simulink model "simulation"  (R2022a)
settings: Solver=VariableStepAuto  StartTime=0.0  StopTime=60  FixedStep=1/1000  RelTol=1e-3
values from neighbouring files (symbols this model uses):
  b = 1    [init.m]
  bw_con = -s_cl    (= 2.66666666667)    [init.m]
  bw_eso = -s_eso    (= 26.6666666667)    [init.m]
  d = 0.1    [init.m]
  eta_init = [0 0 0 0 0]'    [init.m]
  g = 9.82    [init.m]
  L = 1    [init.m]    (also in trig2.m = 1/2 * ((m_c + m_l)*(dx^2 + dy^2 + dz^2) + m_l*L^2*(dtheta^2 )
  ldx_sat = [-5 5]    [init.m]
  ldy_sat = ldx_sat    [init.m]
  ldz_sat = ldx_sat    [init.m]
  m_c = 2.5    [init.m]
  m_l = 0.250    (= 0.25)    [init.m]
  nu_init = [0 0 -L 0 0]'    [init.m]
  xyforce = [-10 10]    [init.m]
  zforce = [-40 40]    [init.m]
libraries: slpidlib x6, SignalEditorBlockLib x1
settings Model: Creator=marti  LastModifiedBy=martin
settings DebuggingCC: UnconnectedInputMsg=warning  UnconnectedOutputMsg=warning  UnconnectedLineMsg=warning
settings RTWCC: DLArmComputeVersion=19.05

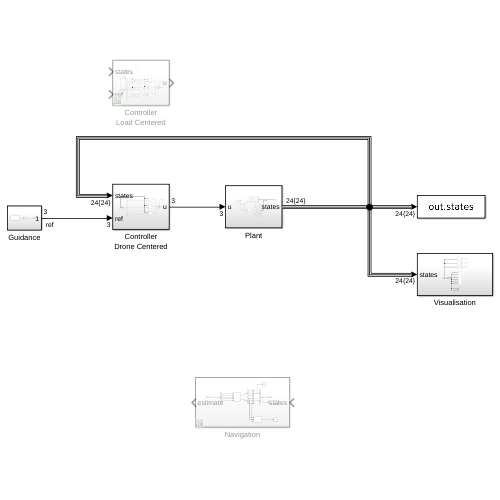
[thumbnail: Simulink's stored preview of the top-level diagram]
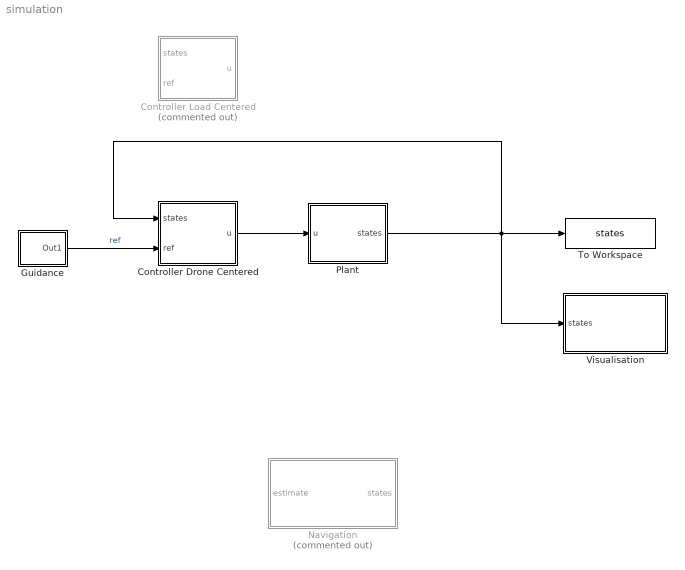
== system simulation ==
  Controller Drone Centered : Subsystem
  Controller Load Centered : Subsystem  Commented=on
  Guidance : Subsystem
  Navigation : Subsystem  Commented=on
  Plant : Subsystem
  To Workspace : ToWorkspace  VariableName=states  SaveFormat=Timeseries  SampleTime=-1
  Visualisation : Subsystem
  wires:
  Plant/1(states) -> Visualisation/1(states), Controller Drone Centered/1(states), To Workspace/1
  Controller Drone Centered/1(u) -> Plant/1(u)
  Guidance/1(Out1) -> Controller Drone Centered/2(ref)  "ref"

== system simulation/Controller Drone Centered ==
  states : Inport
  ref : Inport  Port=2
  Bus Selector : BusSelector  OutputSignals=Quadrotor.vZ
  Bus Selector1 : BusSelector  OutputSignals=Quadrotor.vY
  Bus Selector2 : BusSelector  OutputSignals=Quadrotor.vX
  Bus Selector6 : BusSelector  OutputSignals=Quadrotor.X,Quadrotor.Y,Quadrotor.Z  OutputAsBus=on
  Demux : Demux  Outputs=3
  Forces : Scope
  Mux : Mux  Inputs=3
  PID Controller : slpidlib/PID Controller  Controller=P  Form=Parallel  TimeDomain=Continuous-time  UseExternalTs=off  SampleTime=-1  IntegratorMethod=Forward Euler  FilterMethod=Forward Euler  ControllerParametersSource=internal  P=0.6  I=0  UseKiTs=off  D=0  N=100  UseFilter=on  TunerSelectOption=Transfer Function Based (PID Tuner App)  InitialConditionSource=internal  InitialConditionForIntegrator=0  InitialConditionForFilter=0  DifferentiatorICPrevScaledInput=0  ExternalReset=none  TrackingMode=off  Kt=1  LimitOutput=off  SatLimitsSource=internal  UpperSaturationLimit=inf  LowerSaturationLimit=-inf  LinearizeAsGain=on  AntiWindupMode=none  Kb=1  POutMin=[]  POutMax=[]  IOutMin=[]  IOutMax=[]  DOutMin=[]  DOutMax=[]  NOutMin=[]  NOutMax=[]  SumOutMin=[]  SumOutMax=[]  SaturationOutMin=[]  SaturationOutMax=[]  PParamMin=[]  PParamMax=[]  IParamMin=[]  IParamMax=[]  DParamMin=[]  DParamMax=[]  NParamMin=[]  NParamMax=[]  KbParamMin=[]  KbParamMax=[]  KtParamMin=[]  KtParamMax=[]  KbOutMin=[]  KbOutMax=[]  KtOutMin=[]  KtOutMax=[]  IntegratorOutMin=[]  IntegratorOutMax=[]  FilterOutMin=[]  FilterOutMax=[]  SumI1OutMin=[]  SumI1OutMax=[]  SumI2OutMin=[]  SumI2OutMax=[]  SumI3OutMin=[]  SumI3OutMax=[]  SumI4OutMin=[]  SumI4OutMax=[]  SumDOutMin=[]  SumDOutMax=[]  DifferentiatorOutMin=[]  DifferentiatorOutMax=[]  FilterDiffOutCoefMin=[]  FilterDiffOutCoefMax=[]  ReciprocalOutMin=[]  ReciprocalOutMax=[]  SumDenOutMin=[]  SumDenOutMax=[]  SumNumOutMin=[]  SumNumOutMax=[]  DivideOutMin=[]  DivideOutMax=[]  UdiffTsProdOutMin=[]  UdiffTsProdOutMax=[]  NTsProdOutMin=[]  NTsProdOutMax=[]  UintegralTsProdOutMin=[]  UintegralTsProdOutMax=[]  UngainTsProdOutMin=[]  UngainTsProdOutMax=[]  IntegratorContinuousStateAttributes=''  IntegratorStateMustResolveToSignalObject=off  IntegratorRTWStateStorageClass=Auto  FilterContinuousStateAttributes=''  FilterStateMustResolveToSignalObject=off  FilterRTWStateStorageClass=Auto  ParallelPVariant=InternalParameters  IdealPVariant=Disabled  IVariant=Disabled  DVariant=Disabled  IntegratorVariant=Disabled  SatVariant=Disabled  AWVariant=Disabled  PCopyVariant=Disabled  TRVariant=Disabled  FdbkBlocksVariant=Forward  IdealPFdbkVariant=Disabled  SatFdbkVariant=Disabled  DerivativeFilterVariant=Disabled  NVariant=Disabled  NCopyVariant=Disabled_SignalSpec  FilterICVariant=Disabled  IntegratorICVariant=Disabled  ExternalResetVariant=Disabled  TRSumVariant=Passthrough  SumFdbkVariant=Disabled  SumVariant=Passthrough_P  TsampFilterVariant=InternalTs  TsampNgainVariant=Passthrough  TsampIntegralVariant=Disabled_SignalSpec  ExternalSaturationOutDataTypeStr=Inherit: Same as second input  aMode=0
  PID Controller1 : slpidlib/PID Controller  Controller=P  Form=Parallel  TimeDomain=Continuous-time  UseExternalTs=off  SampleTime=-1  IntegratorMethod=Forward Euler  FilterMethod=Forward Euler  ControllerParametersSource=internal  P=0.6  I=0  UseKiTs=off  D=0  N=100  UseFilter=on  TunerSelectOption=Transfer Function Based (PID Tuner App)  InitialConditionSource=internal  InitialConditionForIntegrator=0  InitialConditionForFilter=0  DifferentiatorICPrevScaledInput=0  ExternalReset=none  TrackingMode=off  Kt=1  LimitOutput=off  SatLimitsSource=internal  UpperSaturationLimit=inf  LowerSaturationLimit=-inf  LinearizeAsGain=on  AntiWindupMode=none  Kb=1  POutMin=[]  POutMax=[]  IOutMin=[]  IOutMax=[]  DOutMin=[]  DOutMax=[]  NOutMin=[]  NOutMax=[]  SumOutMin=[]  SumOutMax=[]  SaturationOutMin=[]  SaturationOutMax=[]  PParamMin=[]  PParamMax=[]  IParamMin=[]  IParamMax=[]  DParamMin=[]  DParamMax=[]  NParamMin=[]  NParamMax=[]  KbParamMin=[]  KbParamMax=[]  KtParamMin=[]  KtParamMax=[]  KbOutMin=[]  KbOutMax=[]  KtOutMin=[]  KtOutMax=[]  IntegratorOutMin=[]  IntegratorOutMax=[]  FilterOutMin=[]  FilterOutMax=[]  SumI1OutMin=[]  SumI1OutMax=[]  SumI2OutMin=[]  SumI2OutMax=[]  SumI3OutMin=[]  SumI3OutMax=[]  SumI4OutMin=[]  SumI4OutMax=[]  SumDOutMin=[]  SumDOutMax=[]  DifferentiatorOutMin=[]  DifferentiatorOutMax=[]  FilterDiffOutCoefMin=[]  FilterDiffOutCoefMax=[]  ReciprocalOutMin=[]  ReciprocalOutMax=[]  SumDenOutMin=[]  SumDenOutMax=[]  SumNumOutMin=[]  SumNumOutMax=[]  DivideOutMin=[]  DivideOutMax=[]  UdiffTsProdOutMin=[]  UdiffTsProdOutMax=[]  NTsProdOutMin=[]  NTsProdOutMax=[]  UintegralTsProdOutMin=[]  UintegralTsProdOutMax=[]  UngainTsProdOutMin=[]  UngainTsProdOutMax=[]  IntegratorContinuousStateAttributes=''  IntegratorStateMustResolveToSignalObject=off  IntegratorRTWStateStorageClass=Auto  FilterContinuousStateAttributes=''  FilterStateMustResolveToSignalObject=off  FilterRTWStateStorageClass=Auto  ParallelPVariant=InternalParameters  IdealPVariant=Disabled  IVariant=Disabled  DVariant=Disabled  IntegratorVariant=Disabled  SatVariant=Disabled  AWVariant=Disabled  PCopyVariant=Disabled  TRVariant=Disabled  FdbkBlocksVariant=Forward  IdealPFdbkVariant=Disabled  SatFdbkVariant=Disabled  DerivativeFilterVariant=Disabled  NVariant=Disabled  NCopyVariant=Disabled_SignalSpec  FilterICVariant=Disabled  IntegratorICVariant=Disabled  ExternalResetVariant=Disabled  TRSumVariant=Passthrough  SumFdbkVariant=Disabled  SumVariant=Passthrough_P  TsampFilterVariant=InternalTs  TsampNgainVariant=Passthrough  TsampIntegralVariant=Disabled_SignalSpec  ExternalSaturationOutDataTypeStr=Inherit: Same as second input  aMode=0
  PID Controller2 : slpidlib/PID Controller  Controller=P  Form=Parallel  TimeDomain=Continuous-time  UseExternalTs=off  SampleTime=-1  IntegratorMethod=Forward Euler  FilterMethod=Forward Euler  ControllerParametersSource=internal  P=0.6  I=0  UseKiTs=off  D=0  N=100  UseFilter=on  TunerSelectOption=Transfer Function Based (PID Tuner App)  InitialConditionSource=internal  InitialConditionForIntegrator=0  InitialConditionForFilter=0  DifferentiatorICPrevScaledInput=0  ExternalReset=none  TrackingMode=off  Kt=1  LimitOutput=off  SatLimitsSource=internal  UpperSaturationLimit=inf  LowerSaturationLimit=-inf  LinearizeAsGain=on  AntiWindupMode=none  Kb=1  POutMin=[]  POutMax=[]  IOutMin=[]  IOutMax=[]  DOutMin=[]  DOutMax=[]  NOutMin=[]  NOutMax=[]  SumOutMin=[]  SumOutMax=[]  SaturationOutMin=[]  SaturationOutMax=[]  PParamMin=[]  PParamMax=[]  IParamMin=[]  IParamMax=[]  DParamMin=[]  DParamMax=[]  NParamMin=[]  NParamMax=[]  KbParamMin=[]  KbParamMax=[]  KtParamMin=[]  KtParamMax=[]  KbOutMin=[]  KbOutMax=[]  KtOutMin=[]  KtOutMax=[]  IntegratorOutMin=[]  IntegratorOutMax=[]  FilterOutMin=[]  FilterOutMax=[]  SumI1OutMin=[]  SumI1OutMax=[]  SumI2OutMin=[]  SumI2OutMax=[]  SumI3OutMin=[]  SumI3OutMax=[]  SumI4OutMin=[]  SumI4OutMax=[]  SumDOutMin=[]  SumDOutMax=[]  DifferentiatorOutMin=[]  DifferentiatorOutMax=[]  FilterDiffOutCoefMin=[]  FilterDiffOutCoefMax=[]  ReciprocalOutMin=[]  ReciprocalOutMax=[]  SumDenOutMin=[]  SumDenOutMax=[]  SumNumOutMin=[]  SumNumOutMax=[]  DivideOutMin=[]  DivideOutMax=[]  UdiffTsProdOutMin=[]  UdiffTsProdOutMax=[]  NTsProdOutMin=[]  NTsProdOutMax=[]  UintegralTsProdOutMin=[]  UintegralTsProdOutMax=[]  UngainTsProdOutMin=[]  UngainTsProdOutMax=[]  IntegratorContinuousStateAttributes=''  IntegratorStateMustResolveToSignalObject=off  IntegratorRTWStateStorageClass=Auto  FilterContinuousStateAttributes=''  FilterStateMustResolveToSignalObject=off  FilterRTWStateStorageClass=Auto  ParallelPVariant=InternalParameters  IdealPVariant=Disabled  IVariant=Disabled  DVariant=Disabled  IntegratorVariant=Disabled  SatVariant=Disabled  AWVariant=Disabled  PCopyVariant=Disabled  TRVariant=Disabled  FdbkBlocksVariant=Forward  IdealPFdbkVariant=Disabled  SatFdbkVariant=Disabled  DerivativeFilterVariant=Disabled  NVariant=Disabled  NCopyVariant=Disabled_SignalSpec  FilterICVariant=Disabled  IntegratorICVariant=Disabled  ExternalResetVariant=Disabled  TRSumVariant=Passthrough  SumFdbkVariant=Disabled  SumVariant=Passthrough_P  TsampFilterVariant=InternalTs  TsampNgainVariant=Passthrough  TsampIntegralVariant=Disabled_SignalSpec  ExternalSaturationOutDataTypeStr=Inherit: Same as second input  aMode=0
  Sum : Sum  Inputs=|-+
  X Velocity LADRC 2nd Order : Subsystem  VariantControl=Choice
  Y Velocity LADRC 2nd Order : Subsystem  VariantControl=Choice
  Z Velocity LADRC 2nd Order : Subsystem  VariantControl=Choice
  u : Outport
  wires:
  Bus Selector/1 -> Z Velocity LADRC 2nd Order/1(y)  "<vZ>"
  states/1 -> Bus Selector6/1, Bus Selector/1, Bus Selector1/1, Bus Selector2/1
  Y Velocity LADRC 2nd Order/1(u) -> Mux/2  "f_y"
  Z Velocity LADRC 2nd Order/1(u) -> Mux/3  "f_z"
  PID Controller/1 -> X Velocity LADRC 2nd Order/2(r)  "f_x"
  Bus Selector1/1 -> Y Velocity LADRC 2nd Order/1(y)  "<vY>"
  Bus Selector2/1 -> X Velocity LADRC 2nd Order/1(y)  "<vX>"
  Mux/1 -> Forces/1, u/1
  Bus Selector6/1 -> Sum/1
  ref/1 -> Sum/2
  Sum/1 -> Demux/1
  PID Controller2/1 -> Z Velocity LADRC 2nd Order/2(r)  "f_x"
  X Velocity LADRC 2nd Order/1(u) -> Mux/1  "f_x"
  PID Controller1/1 -> Y Velocity LADRC 2nd Order/2(r)
  Demux/1 -> PID Controller/1
  Demux/2 -> PID Controller1/1
  Demux/3 -> PID Controller2/1

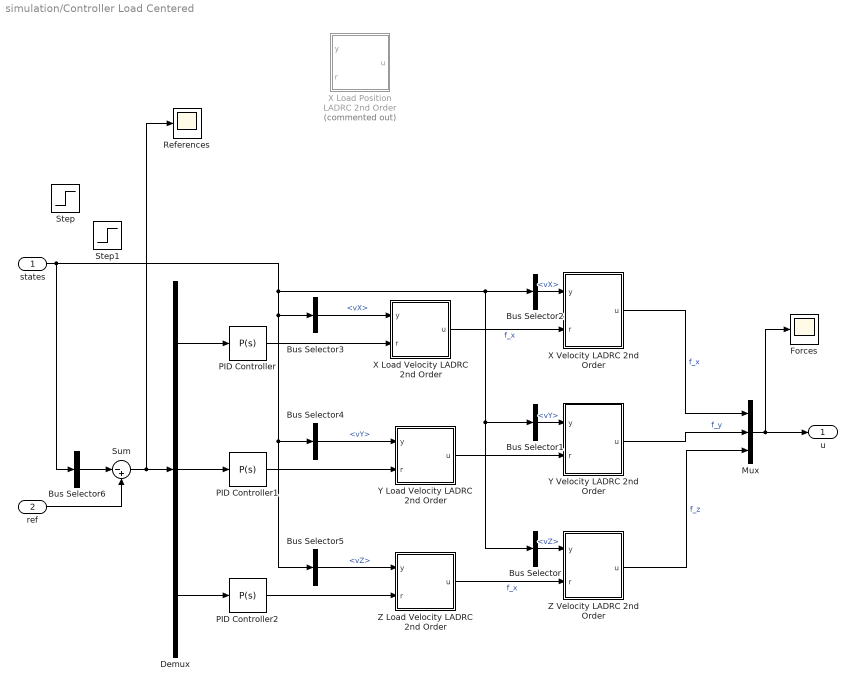
== system simulation/Controller Load Centered ==
  states : Inport
  ref : Inport  Port=2
  Bus Selector : BusSelector  OutputSignals=Quadrotor.vZ
  Bus Selector1 : BusSelector  OutputSignals=Quadrotor.vY
  Bus Selector2 : BusSelector  OutputSignals=Quadrotor.vX
  Bus Selector3 : BusSelector  OutputSignals=Load.vX
  Bus Selector4 : BusSelector  OutputSignals=Load.vY
  Bus Selector5 : BusSelector  OutputSignals=Load.vZ
  Bus Selector6 : BusSelector  OutputSignals=Load.X,Load.Y,Load.Z  OutputAsBus=on
  Demux : Demux  Outputs=3
  Forces : Scope
  Mux : Mux  Inputs=3
  PID Controller : slpidlib/PID Controller  Controller=P  Form=Parallel  TimeDomain=Continuous-time  UseExternalTs=off  SampleTime=-1  IntegratorMethod=Forward Euler  FilterMethod=Forward Euler  ControllerParametersSource=internal  P=0.6  I=0  UseKiTs=off  D=0  N=100  UseFilter=on  TunerSelectOption=Transfer Function Based (PID Tuner App)  InitialConditionSource=internal  InitialConditionForIntegrator=0  InitialConditionForFilter=0  DifferentiatorICPrevScaledInput=0  ExternalReset=none  TrackingMode=off  Kt=1  LimitOutput=off  SatLimitsSource=internal  UpperSaturationLimit=inf  LowerSaturationLimit=-inf  LinearizeAsGain=on  AntiWindupMode=none  Kb=1  POutMin=[]  POutMax=[]  IOutMin=[]  IOutMax=[]  DOutMin=[]  DOutMax=[]  NOutMin=[]  NOutMax=[]  SumOutMin=[]  SumOutMax=[]  SaturationOutMin=[]  SaturationOutMax=[]  PParamMin=[]  PParamMax=[]  IParamMin=[]  IParamMax=[]  DParamMin=[]  DParamMax=[]  NParamMin=[]  NParamMax=[]  KbParamMin=[]  KbParamMax=[]  KtParamMin=[]  KtParamMax=[]  KbOutMin=[]  KbOutMax=[]  KtOutMin=[]  KtOutMax=[]  IntegratorOutMin=[]  IntegratorOutMax=[]  FilterOutMin=[]  FilterOutMax=[]  SumI1OutMin=[]  SumI1OutMax=[]  SumI2OutMin=[]  SumI2OutMax=[]  SumI3OutMin=[]  SumI3OutMax=[]  SumI4OutMin=[]  SumI4OutMax=[]  SumDOutMin=[]  SumDOutMax=[]  DifferentiatorOutMin=[]  DifferentiatorOutMax=[]  FilterDiffOutCoefMin=[]  FilterDiffOutCoefMax=[]  ReciprocalOutMin=[]  ReciprocalOutMax=[]  SumDenOutMin=[]  SumDenOutMax=[]  SumNumOutMin=[]  SumNumOutMax=[]  DivideOutMin=[]  DivideOutMax=[]  UdiffTsProdOutMin=[]  UdiffTsProdOutMax=[]  NTsProdOutMin=[]  NTsProdOutMax=[]  UintegralTsProdOutMin=[]  UintegralTsProdOutMax=[]  UngainTsProdOutMin=[]  UngainTsProdOutMax=[]  IntegratorContinuousStateAttributes=''  IntegratorStateMustResolveToSignalObject=off  IntegratorRTWStateStorageClass=Auto  FilterContinuousStateAttributes=''  FilterStateMustResolveToSignalObject=off  FilterRTWStateStorageClass=Auto  ParallelPVariant=InternalParameters  IdealPVariant=Disabled  IVariant=Disabled  DVariant=Disabled  IntegratorVariant=Disabled  SatVariant=Disabled  AWVariant=Disabled  PCopyVariant=Disabled  TRVariant=Disabled  FdbkBlocksVariant=Forward  IdealPFdbkVariant=Disabled  SatFdbkVariant=Disabled  DerivativeFilterVariant=Disabled  NVariant=Disabled  NCopyVariant=Disabled_SignalSpec  FilterICVariant=Disabled  IntegratorICVariant=Disabled  ExternalResetVariant=Disabled  TRSumVariant=Passthrough  SumFdbkVariant=Disabled  SumVariant=Passthrough_P  TsampFilterVariant=InternalTs  TsampNgainVariant=Passthrough  TsampIntegralVariant=Disabled_SignalSpec  ExternalSaturationOutDataTypeStr=Inherit: Same as second input  aMode=0
  PID Controller1 : slpidlib/PID Controller  Controller=P  Form=Parallel  TimeDomain=Continuous-time  UseExternalTs=off  SampleTime=-1  IntegratorMethod=Forward Euler  FilterMethod=Forward Euler  ControllerParametersSource=internal  P=0.6  I=0  UseKiTs=off  D=0  N=100  UseFilter=on  TunerSelectOption=Transfer Function Based (PID Tuner App)  InitialConditionSource=internal  InitialConditionForIntegrator=0  InitialConditionForFilter=0  DifferentiatorICPrevScaledInput=0  ExternalReset=none  TrackingMode=off  Kt=1  LimitOutput=off  SatLimitsSource=internal  UpperSaturationLimit=inf  LowerSaturationLimit=-inf  LinearizeAsGain=on  AntiWindupMode=none  Kb=1  POutMin=[]  POutMax=[]  IOutMin=[]  IOutMax=[]  DOutMin=[]  DOutMax=[]  NOutMin=[]  NOutMax=[]  SumOutMin=[]  SumOutMax=[]  SaturationOutMin=[]  SaturationOutMax=[]  PParamMin=[]  PParamMax=[]  IParamMin=[]  IParamMax=[]  DParamMin=[]  DParamMax=[]  NParamMin=[]  NParamMax=[]  KbParamMin=[]  KbParamMax=[]  KtParamMin=[]  KtParamMax=[]  KbOutMin=[]  KbOutMax=[]  KtOutMin=[]  KtOutMax=[]  IntegratorOutMin=[]  IntegratorOutMax=[]  FilterOutMin=[]  FilterOutMax=[]  SumI1OutMin=[]  SumI1OutMax=[]  SumI2OutMin=[]  SumI2OutMax=[]  SumI3OutMin=[]  SumI3OutMax=[]  SumI4OutMin=[]  SumI4OutMax=[]  SumDOutMin=[]  SumDOutMax=[]  DifferentiatorOutMin=[]  DifferentiatorOutMax=[]  FilterDiffOutCoefMin=[]  FilterDiffOutCoefMax=[]  ReciprocalOutMin=[]  ReciprocalOutMax=[]  SumDenOutMin=[]  SumDenOutMax=[]  SumNumOutMin=[]  SumNumOutMax=[]  DivideOutMin=[]  DivideOutMax=[]  UdiffTsProdOutMin=[]  UdiffTsProdOutMax=[]  NTsProdOutMin=[]  NTsProdOutMax=[]  UintegralTsProdOutMin=[]  UintegralTsProdOutMax=[]  UngainTsProdOutMin=[]  UngainTsProdOutMax=[]  IntegratorContinuousStateAttributes=''  IntegratorStateMustResolveToSignalObject=off  IntegratorRTWStateStorageClass=Auto  FilterContinuousStateAttributes=''  FilterStateMustResolveToSignalObject=off  FilterRTWStateStorageClass=Auto  ParallelPVariant=InternalParameters  IdealPVariant=Disabled  IVariant=Disabled  DVariant=Disabled  IntegratorVariant=Disabled  SatVariant=Disabled  AWVariant=Disabled  PCopyVariant=Disabled  TRVariant=Disabled  FdbkBlocksVariant=Forward  IdealPFdbkVariant=Disabled  SatFdbkVariant=Disabled  DerivativeFilterVariant=Disabled  NVariant=Disabled  NCopyVariant=Disabled_SignalSpec  FilterICVariant=Disabled  IntegratorICVariant=Disabled  ExternalResetVariant=Disabled  TRSumVariant=Passthrough  SumFdbkVariant=Disabled  SumVariant=Passthrough_P  TsampFilterVariant=InternalTs  TsampNgainVariant=Passthrough  TsampIntegralVariant=Disabled_SignalSpec  ExternalSaturationOutDataTypeStr=Inherit: Same as second input  aMode=0
  PID Controller2 : slpidlib/PID Controller  Controller=P  Form=Parallel  TimeDomain=Continuous-time  UseExternalTs=off  SampleTime=-1  IntegratorMethod=Forward Euler  FilterMethod=Forward Euler  ControllerParametersSource=internal  P=0.6  I=0  UseKiTs=off  D=0  N=100  UseFilter=on  TunerSelectOption=Transfer Function Based (PID Tuner App)  InitialConditionSource=internal  InitialConditionForIntegrator=0  InitialConditionForFilter=0  DifferentiatorICPrevScaledInput=0  ExternalReset=none  TrackingMode=off  Kt=1  LimitOutput=off  SatLimitsSource=internal  UpperSaturationLimit=inf  LowerSaturationLimit=-inf  LinearizeAsGain=on  AntiWindupMode=none  Kb=1  POutMin=[]  POutMax=[]  IOutMin=[]  IOutMax=[]  DOutMin=[]  DOutMax=[]  NOutMin=[]  NOutMax=[]  SumOutMin=[]  SumOutMax=[]  SaturationOutMin=[]  SaturationOutMax=[]  PParamMin=[]  PParamMax=[]  IParamMin=[]  IParamMax=[]  DParamMin=[]  DParamMax=[]  NParamMin=[]  NParamMax=[]  KbParamMin=[]  KbParamMax=[]  KtParamMin=[]  KtParamMax=[]  KbOutMin=[]  KbOutMax=[]  KtOutMin=[]  KtOutMax=[]  IntegratorOutMin=[]  IntegratorOutMax=[]  FilterOutMin=[]  FilterOutMax=[]  SumI1OutMin=[]  SumI1OutMax=[]  SumI2OutMin=[]  SumI2OutMax=[]  SumI3OutMin=[]  SumI3OutMax=[]  SumI4OutMin=[]  SumI4OutMax=[]  SumDOutMin=[]  SumDOutMax=[]  DifferentiatorOutMin=[]  DifferentiatorOutMax=[]  FilterDiffOutCoefMin=[]  FilterDiffOutCoefMax=[]  ReciprocalOutMin=[]  ReciprocalOutMax=[]  SumDenOutMin=[]  SumDenOutMax=[]  SumNumOutMin=[]  SumNumOutMax=[]  DivideOutMin=[]  DivideOutMax=[]  UdiffTsProdOutMin=[]  UdiffTsProdOutMax=[]  NTsProdOutMin=[]  NTsProdOutMax=[]  UintegralTsProdOutMin=[]  UintegralTsProdOutMax=[]  UngainTsProdOutMin=[]  UngainTsProdOutMax=[]  IntegratorContinuousStateAttributes=''  IntegratorStateMustResolveToSignalObject=off  IntegratorRTWStateStorageClass=Auto  FilterContinuousStateAttributes=''  FilterStateMustResolveToSignalObject=off  FilterRTWStateStorageClass=Auto  ParallelPVariant=InternalParameters  IdealPVariant=Disabled  IVariant=Disabled  DVariant=Disabled  IntegratorVariant=Disabled  SatVariant=Disabled  AWVariant=Disabled  PCopyVariant=Disabled  TRVariant=Disabled  FdbkBlocksVariant=Forward  IdealPFdbkVariant=Disabled  SatFdbkVariant=Disabled  DerivativeFilterVariant=Disabled  NVariant=Disabled  NCopyVariant=Disabled_SignalSpec  FilterICVariant=Disabled  IntegratorICVariant=Disabled  ExternalResetVariant=Disabled  TRSumVariant=Passthrough  SumFdbkVariant=Disabled  SumVariant=Passthrough_P  TsampFilterVariant=InternalTs  TsampNgainVariant=Passthrough  TsampIntegralVariant=Disabled_SignalSpec  ExternalSaturationOutDataTypeStr=Inherit: Same as second input  aMode=0
  References : Scope
  Step : Step  Time=5  After=4  SampleTime=0
  Step1 : Step  Time=10  After=4  SampleTime=0
  Sum : Sum  Inputs=|-+
  X Load Position LADRC 2nd Order : Subsystem  Commented=on  VariantControl=Choice
  X Load Velocity LADRC 2nd Order : Subsystem  VariantControl=Choice
  X Velocity LADRC 2nd Order : Subsystem  VariantControl=Choice
  Y Load Velocity LADRC 2nd Order : Subsystem  VariantControl=Choice
  Y Velocity LADRC 2nd Order : Subsystem  VariantControl=Choice
  Z Load Velocity LADRC 2nd Order : Subsystem  VariantControl=Choice
  Z Velocity LADRC 2nd Order : Subsystem  VariantControl=Choice
  u : Outport
  wires:
  Bus Selector/1 -> Z Velocity LADRC 2nd Order/1(y)  "<vZ>"
  states/1 -> Bus Selector6/1, Bus Selector5/1, Bus Selector4/1, Bus Selector3/1, Bus Selector/1, Bus Selector1/1, Bus Selector2/1
  Y Velocity LADRC 2nd Order/1(u) -> Mux/2  "f_y"
  Z Velocity LADRC 2nd Order/1(u) -> Mux/3  "f_z"
  X Load Velocity LADRC 2nd Order/1(u) -> X Velocity LADRC 2nd Order/2(r)  "f_x"
  Bus Selector1/1 -> Y Velocity LADRC 2nd Order/1(y)  "<vY>"
  Bus Selector2/1 -> X Velocity LADRC 2nd Order/1(y)  "<vX>"
  Mux/1 -> Forces/1, u/1
  Bus Selector3/1 -> X Load Velocity LADRC 2nd Order/1(y)  "<vX>"
  Bus Selector4/1 -> Y Load Velocity LADRC 2nd Order/1(y)  "<vY>"
  Bus Selector5/1 -> Z Load Velocity LADRC 2nd Order/1(y)  "<vZ>"
  Bus Selector6/1 -> Sum/1
  ref/1 -> Sum/2
  Sum/1 -> References/1, Demux/1
  Z Load Velocity LADRC 2nd Order/1(u) -> Z Velocity LADRC 2nd Order/2(r)  "f_x"
  X Velocity LADRC 2nd Order/1(u) -> Mux/1  "f_x"
  Y Load Velocity LADRC 2nd Order/1(u) -> Y Velocity LADRC 2nd Order/2(r)
  PID Controller/1 -> X Load Velocity LADRC 2nd Order/2(r)
  PID Controller2/1 -> Z Load Velocity LADRC 2nd Order/2(r)
  PID Controller1/1 -> Y Load Velocity LADRC 2nd Order/2(r)
  Demux/1 -> PID Controller/1
  Demux/2 -> PID Controller1/1
  Demux/3 -> PID Controller2/1

== system simulation/Guidance ==
  Gain : Gain
  Signal Editor : SignalEditorBlockLib/Signal Editor  FileName=trajectories.mat  ActiveScenario=Load_Steps  ActiveSignal=Signal  IsBus=off  OutputBusObjectStr=Bus: BusObject  SampleTime=0  Interpolate=off  ZeroCross=off  OutputAfterFinalValue=Setting to zero  Unit=inherit  PreserveSignalName=on
  Out1 : Outport
  wires:
  Signal Editor/1 -> Gain/1
  Gain/1 -> Out1/1

== system simulation/Navigation ==
  states : Inport
  Bus Creator : BusCreator  Inputs=3
  Bus Creator1 : BusCreator  Inputs=3
  Bus Creator2 : BusCreator  Inputs=2
  Bus Selector : BusSelector  OutputSignals=Position.X,Position.Y,Position.Z,Position.Phi,Position.Theta
  Demux : Demux  Outputs=3
  Demux1 : Demux  Outputs=3
  Load Position : Scope
  MATLAB Function : MATLAB Function  TreatAsAtomicUnit=on
  MATLAB Function1 : MATLAB Function  TreatAsAtomicUnit=on
  Scope : Scope
  To Workspace : ToWorkspace  VariableName=estimate  SaveFormat=Timeseries  SampleTime=-1
  estimate : Outport
  wires:
  states/1 -> Bus Selector/1
  Bus Selector/1 -> MATLAB Function/1(x)  "<X>"
  Bus Selector/2 -> MATLAB Function/2(y)  "<Y>"
  Bus Selector/3 -> MATLAB Function/3(z)  "<Z>"
  Bus Selector/4 -> MATLAB Function/4(phi)  "<Phi>"
  Bus Selector/5 -> MATLAB Function/5(theta)  "<Theta>"
  MATLAB Function/1(pos) -> Demux/1
  Demux/1 -> Bus Creator/1  "X"
  Demux/2 -> Bus Creator/2  "Y"
  Demux/3 -> Bus Creator/3  "Z"
  Demux1/1 -> MATLAB Function1/2(y), Bus Creator1/1  "X"
  MATLAB Function/2(vect) -> Demux1/1
  Demux1/2 -> MATLAB Function1/1(x), Bus Creator1/2  "Y"
  Demux1/3 -> MATLAB Function1/3(z), Bus Creator1/3  "Z"
  Bus Creator/1 -> Load Position/1, Bus Creator2/1  "Position"
  Bus Creator1/1 -> Bus Creator2/2  "Vector"
  Bus Creator2/1 -> To Workspace/1, estimate/1
  MATLAB Function1/1(norm) -> Scope/1

== system simulation/Plant ==
  u : Inport
  Bus Creator : BusCreator  Inputs=15
  Bus Creator1 : BusCreator  Inputs=2
  Bus Creator4 : BusCreator  Inputs=9
  Demux : Demux  Outputs=5
  Demux1 : Demux  Outputs=5
  Demux2 : Demux  Outputs=5
  Demux3 : Demux  Outputs=3
  Demux4 : Demux  Outputs=3
  Demux5 : Demux  Outputs=3
  Integrator : Integrator  InitialCondition=eta_init
  Integrator1 : Integrator  InitialCondition=nu_init
  Load Polar to Cartesian : MATLAB Function  TreatAsAtomicUnit=on
  MATLAB Function : MATLAB Function  TreatAsAtomicUnit=on
  Selector : Selector  InputPortWidth=5  IndexOptions=Index vector (dialog)  Indices=[1 2 3]  OutputSizes=1
  Selector1 : Selector  InputPortWidth=5  IndexOptions=Index vector (dialog)  Indices=[1 2 3]  OutputSizes=1
  Selector2 : Selector  InputPortWidth=5  IndexOptions=Index vector (dialog)  Indices=[1 2 3]  OutputSizes=1
  states : Outport
  wires:
  Integrator/1 -> Selector1/1, Load Polar to Cartesian/2(qd), MATLAB Function/2(eta), Integrator1/1  "eta"
  MATLAB Function/1(eta_d) -> Load Polar to Cartesian/3(qdd), Integrator/1, Selector2/1
  u/1 -> MATLAB Function/3(u)
  Integrator1/1 -> Selector/1, Load Polar to Cartesian/1(q), MATLAB Function/1(nu)  "nu"
  Bus Creator1/1 -> states/1
  Selector/1 -> Demux3/1
  Selector1/1 -> Demux4/1
  Selector2/1 -> Demux5/1
  Demux3/1 -> Bus Creator4/1  "X"
  Demux3/2 -> Bus Creator4/2  "Y"
  Demux3/3 -> Bus Creator4/3  "Z"
  Demux4/1 -> Bus Creator4/4  "vX"
  Demux4/2 -> Bus Creator4/5  "vY"
  Demux4/3 -> Bus Creator4/6  "vZ"
  Demux5/1 -> Bus Creator4/7  "aX"
  Demux5/2 -> Bus Creator4/8  "aY"
  Demux5/3 -> Bus Creator4/9  "aZ"
  Bus Creator4/1 -> Bus Creator1/1  "Quadrotor"
  Load Polar to Cartesian/1(pos) -> Demux/1
  Load Polar to Cartesian/2(vel) -> Demux1/1
  Load Polar to Cartesian/3(acc) -> Demux2/1
  Demux/1 -> Bus Creator/1  "X"
  Demux/2 -> Bus Creator/2  "Y"
  Demux/3 -> Bus Creator/3  "Z"
  Demux/4 -> Bus Creator/4  "Theta"
  Demux/5 -> Bus Creator/5  "Phi"
  Demux1/1 -> Bus Creator/6  "vX"
  Demux1/2 -> Bus Creator/7  "vY"
  Demux1/3 -> Bus Creator/8  "vZ"
  Demux1/4 -> Bus Creator/9  "vTheta"
  Demux1/5 -> Bus Creator/10  "vPhi"
  Demux2/1 -> Bus Creator/11  "aX"
  Demux2/2 -> Bus Creator/12  "aY"
  Demux2/3 -> Bus Creator/13  "aZ"
  Demux2/4 -> Bus Creator/14  "aTheta"
  Demux2/5 -> Bus Creator/15  "aPhi"
  Bus Creator/1 -> Bus Creator1/2  "Load"

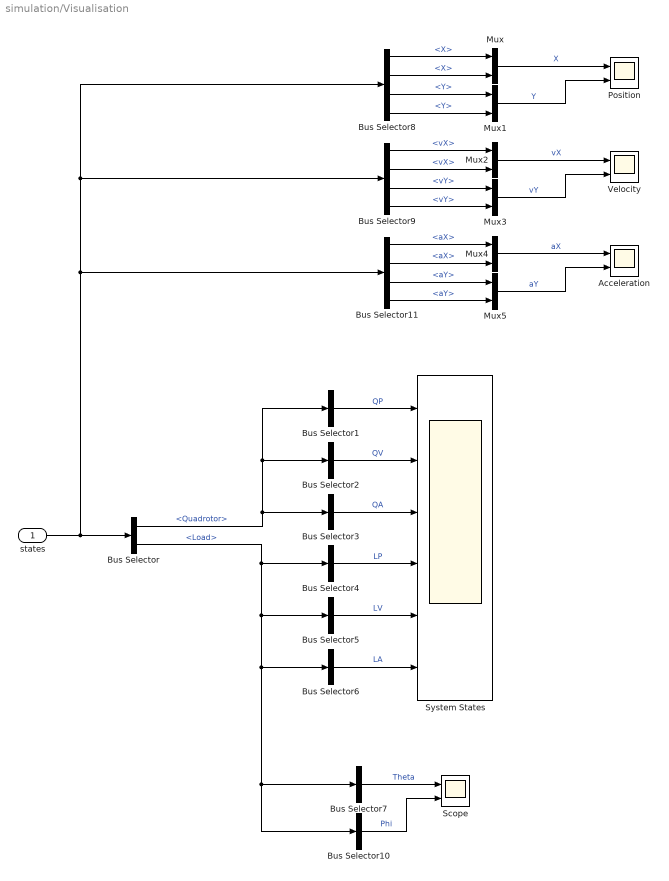
== system simulation/Visualisation ==
  states : Inport
  Acceleration : Scope  NumInputPorts=2
  Bus Selector : BusSelector  OutputSignals=Quadrotor,Load
  Bus Selector1 : BusSelector  OutputSignals=X,Y,Z  OutputAsBus=on
  Bus Selector10 : BusSelector  OutputSignals=Phi,vPhi,aPhi  OutputAsBus=on
  Bus Selector11 : BusSelector  OutputSignals=Quadrotor.aX,Load.aX,Quadrotor.aY,Load.aY
  Bus Selector2 : BusSelector  OutputSignals=vX,vY,vZ  OutputAsBus=on
  Bus Selector3 : BusSelector  OutputSignals=aX,aY,aZ  OutputAsBus=on
  Bus Selector4 : BusSelector  OutputSignals=X,Y,Z  OutputAsBus=on
  Bus Selector5 : BusSelector  OutputSignals=vX,vY,vZ  OutputAsBus=on
  Bus Selector6 : BusSelector  OutputSignals=aX,aY,aZ  OutputAsBus=on
  Bus Selector7 : BusSelector  OutputSignals=Theta,vTheta,aTheta  OutputAsBus=on
  Bus Selector8 : BusSelector  OutputSignals=Quadrotor.X,Load.X,Quadrotor.Y,Load.Y
  Bus Selector9 : BusSelector  OutputSignals=Quadrotor.vX,Load.vX,Quadrotor.vY,Load.vY
  Mux{,1..5} (6 alike) : Mux  Inputs=2
  Position : Scope  NumInputPorts=2
  Scope : Scope  NumInputPorts=2
  System States : Scope  NumInputPorts=6
  Velocity : Scope  NumInputPorts=2
  wires:
  Bus Selector/1 -> Bus Selector1/1, Bus Selector2/1, Bus Selector3/1  "<Quadrotor>"
  Bus Selector1/1 -> System States/1  "QP"
  Bus Selector2/1 -> System States/2  "QV"
  Bus Selector3/1 -> System States/3  "QA"
  Bus Selector4/1 -> System States/4  "LP"
  Bus Selector5/1 -> System States/5  "LV"
  Bus Selector6/1 -> System States/6  "LA"
  Bus Selector/2 -> Bus Selector10/1, Bus Selector7/1, Bus Selector6/1, Bus Selector5/1, Bus Selector4/1  "<Load>"
  Bus Selector7/1 -> Scope/1  "Theta"
  Bus Selector8/1 -> Mux/1  "<X>"
  Bus Selector8/2 -> Mux/2  "<X>"
  Mux/1 -> Position/1  "X"
  Bus Selector8/3 -> Mux1/1  "<Y>"
  Bus Selector8/4 -> Mux1/2  "<Y>"
  Mux1/1 -> Position/2  "Y"
  Bus Selector9/2 -> Mux2/2  "<vX>"
  Mux2/1 -> Velocity/1  "vX"
  Bus Selector9/4 -> Mux3/2  "<vY>"
  Bus Selector9/3 -> Mux3/1  "<vY>"
  Bus Selector9/1 -> Mux2/1  "<vX>"
  Mux3/1 -> Velocity/2  "vY"
  Bus Selector10/1 -> Scope/2  "Phi"
  Mux5/1 -> Acceleration/2  "aY"
  Mux4/1 -> Acceleration/1  "aX"
  Bus Selector11/3 -> Mux5/1  "<aY>"
  Bus Selector11/2 -> Mux4/2  "<aX>"
  states/1 -> Bus Selector11/1, Bus Selector9/1, Bus Selector8/1, Bus Selector/1
  Bus Selector11/1 -> Mux4/1  "<aX>"
  Bus Selector11/4 -> Mux5/2  "<aY>"

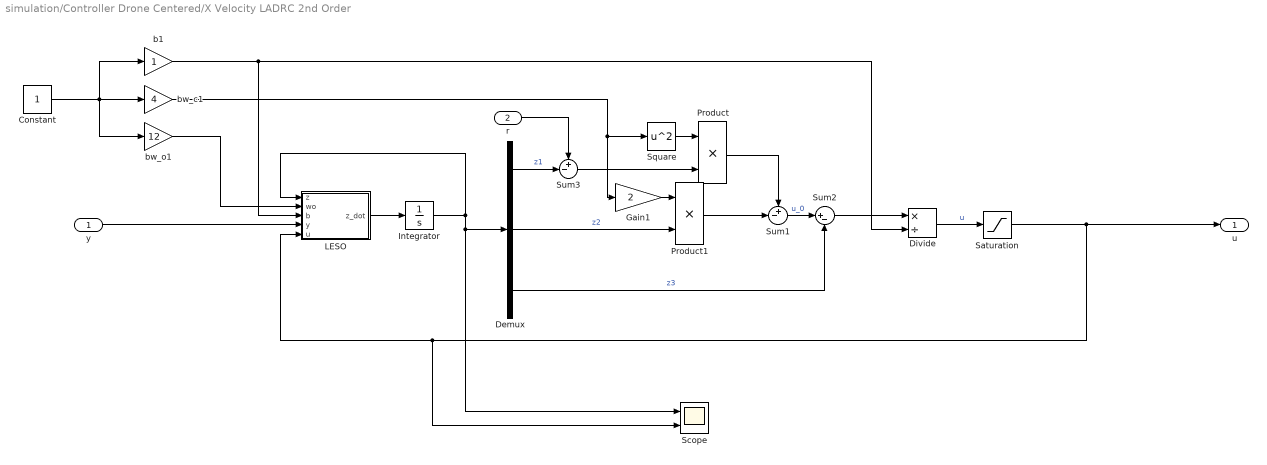
== system simulation/Controller Drone Centered/X Velocity LADRC 2nd Order ==
  y : Inport
  r : Inport  Port=2
  Constant : Constant
  Demux : Demux  Outputs=3
  Divide : Product  Inputs=*/
  Gain1 : Gain  Gain=2
  Integrator : Integrator  InitialCondition=[0 0 0]'
  LESO : MATLAB Function  TreatAsAtomicUnit=on
  Product : Product
  Product1 : Product
  Saturation : Saturate  UpperLimit=xyforce(2)  LowerLimit=xyforce(1)
  Scope : Scope  NumInputPorts=2
  Square : Math  Operator=square
  Sum1 : Sum  Inputs=+-|
  Sum2 : Sum  Inputs=|+-
  Sum3 : Sum  Inputs=+-|
  b1 : Gain
  bw_c1 : Gain  Gain=4
  bw_o1 : Gain  Gain=12
  u : Outport
  wires:
  LESO/1(z_dot) -> Integrator/1
  Integrator/1 -> LESO/1(z), Scope/1, Demux/1
  Demux/1 -> Sum3/2  "z1"
  Product/1 -> Sum1/1
  Sum1/1 -> Sum2/1  "u_0"
  Demux/3 -> Sum2/2  "z3"
  Sum2/1 -> Divide/1
  Square/1 -> Product/1
  Gain1/1 -> Product1/1
  Demux/2 -> Product1/2  "z2"
  Product1/1 -> Sum1/2
  r/1 -> Sum3/1
  Sum3/1 -> Product/2
  b1/1 -> Divide/2, LESO/3(b)
  bw_c1/1 -> Gain1/1, Square/1
  bw_o1/1 -> LESO/2(wo)
  y/1 -> LESO/4(y)
  Constant/1 -> bw_o1/1, bw_c1/1, b1/1
  Divide/1 -> Saturation/1  "u"
  Saturation/1 -> Scope/2, LESO/5(u), u/1

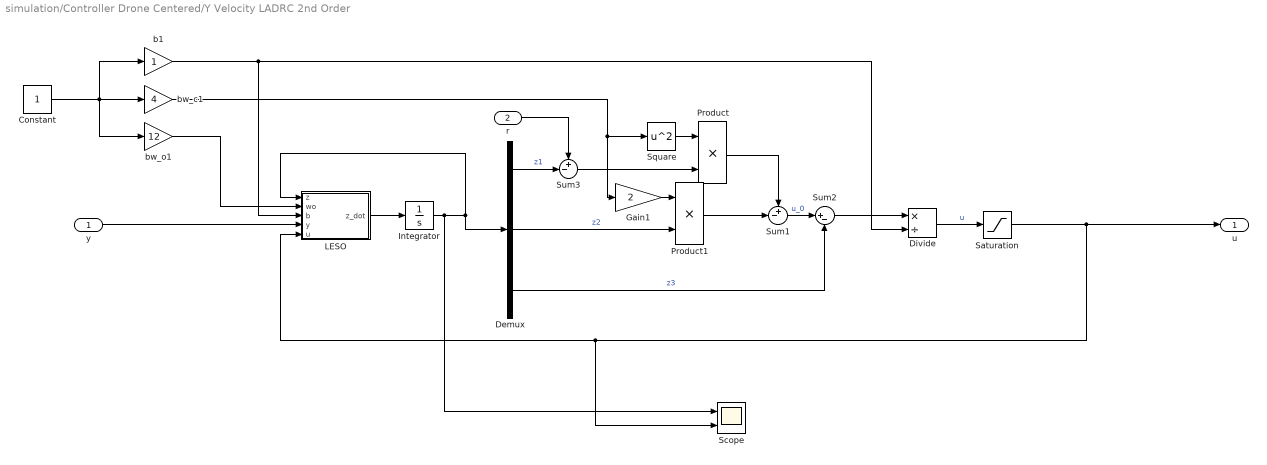
== system simulation/Controller Drone Centered/Y Velocity LADRC 2nd Order ==
  y : Inport
  r : Inport  Port=2
  Constant : Constant
  Demux : Demux  Outputs=3
  Divide : Product  Inputs=*/
  Gain1 : Gain  Gain=2
  Integrator : Integrator  InitialCondition=[0 0 0]'
  LESO : MATLAB Function  TreatAsAtomicUnit=on
  Product : Product
  Product1 : Product
  Saturation : Saturate  UpperLimit=xyforce(2)  LowerLimit=xyforce(1)
  Scope : Scope  NumInputPorts=2
  Square : Math  Operator=square
  Sum1 : Sum  Inputs=+-|
  Sum2 : Sum  Inputs=|+-
  Sum3 : Sum  Inputs=+-|
  b1 : Gain
  bw_c1 : Gain  Gain=4
  bw_o1 : Gain  Gain=12
  u : Outport
  wires:
  LESO/1(z_dot) -> Integrator/1
  Integrator/1 -> Scope/1, LESO/1(z), Demux/1
  Demux/1 -> Sum3/2  "z1"
  Product/1 -> Sum1/1
  Sum1/1 -> Sum2/1  "u_0"
  Demux/3 -> Sum2/2  "z3"
  Sum2/1 -> Divide/1
  Square/1 -> Product/1
  Gain1/1 -> Product1/1
  Demux/2 -> Product1/2  "z2"
  Product1/1 -> Sum1/2
  r/1 -> Sum3/1
  Sum3/1 -> Product/2
  b1/1 -> Divide/2, LESO/3(b)
  bw_c1/1 -> Gain1/1, Square/1
  bw_o1/1 -> LESO/2(wo)
  y/1 -> LESO/4(y)
  Constant/1 -> bw_o1/1, bw_c1/1, b1/1
  Divide/1 -> Saturation/1  "u"
  Saturation/1 -> Scope/2, LESO/5(u), u/1

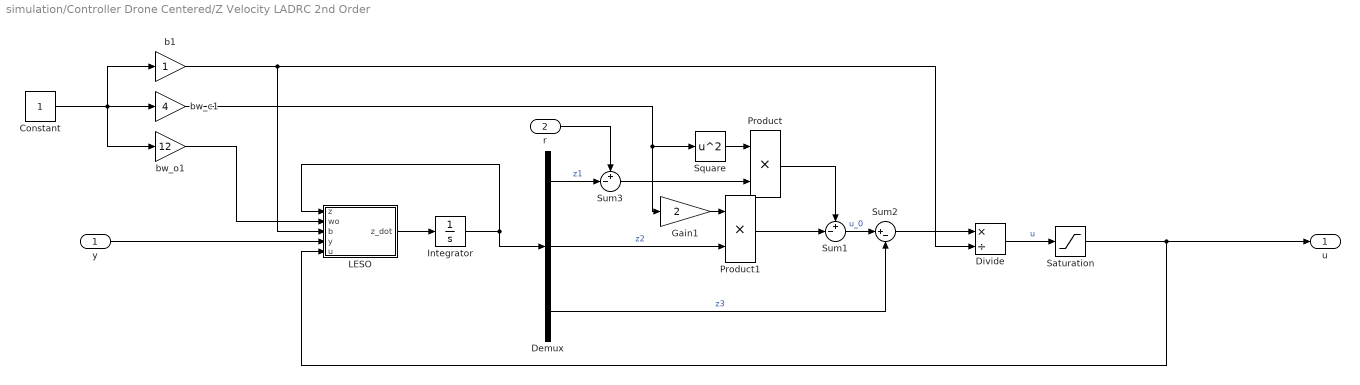
== system simulation/Controller Drone Centered/Z Velocity LADRC 2nd Order ==
  y : Inport
  r : Inport  Port=2
  Constant : Constant
  Demux : Demux  Outputs=3
  Divide : Product  Inputs=*/
  Gain1 : Gain  Gain=2
  Integrator : Integrator  InitialCondition=[0 0 0]'
  LESO : MATLAB Function  TreatAsAtomicUnit=on
  Product : Product
  Product1 : Product
  Saturation : Saturate  UpperLimit=zforce(2)  LowerLimit=zforce(1)
  Square : Math  Operator=square
  Sum1 : Sum  Inputs=+-|
  Sum2 : Sum  Inputs=|+-
  Sum3 : Sum  Inputs=+-|
  b1 : Gain
  bw_c1 : Gain  Gain=4
  bw_o1 : Gain  Gain=12
  u : Outport
  wires:
  LESO/1(z_dot) -> Integrator/1
  Integrator/1 -> LESO/1(z), Demux/1
  Demux/1 -> Sum3/2  "z1"
  Product/1 -> Sum1/1
  Sum1/1 -> Sum2/1  "u_0"
  Demux/3 -> Sum2/2  "z3"
  Sum2/1 -> Divide/1
  Square/1 -> Product/1
  Gain1/1 -> Product1/1
  Demux/2 -> Product1/2  "z2"
  Product1/1 -> Sum1/2
  r/1 -> Sum3/1
  Sum3/1 -> Product/2
  b1/1 -> Divide/2, LESO/3(b)
  bw_c1/1 -> Gain1/1, Square/1
  bw_o1/1 -> LESO/2(wo)
  y/1 -> LESO/4(y)
  Constant/1 -> bw_o1/1, bw_c1/1, b1/1
  Divide/1 -> Saturation/1  "u"
  Saturation/1 -> LESO/5(u), u/1

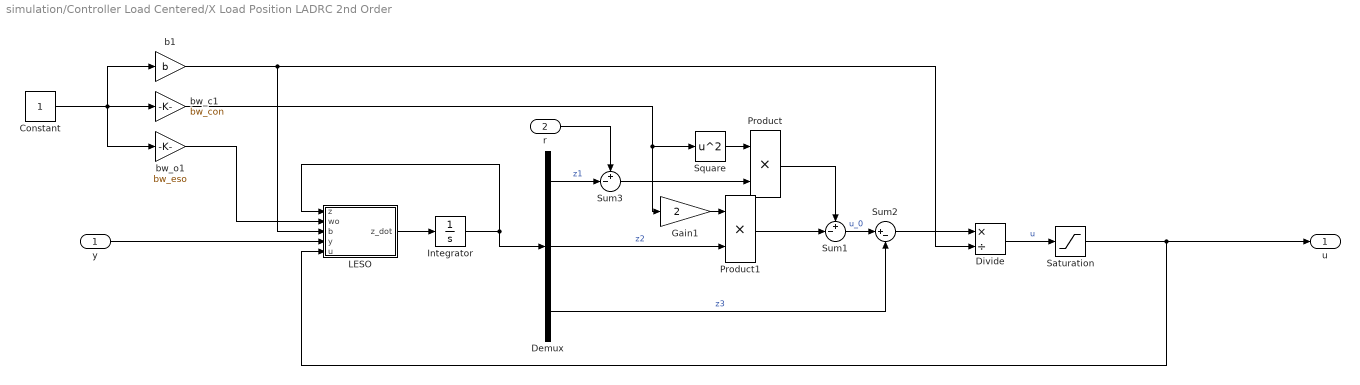
== system simulation/Controller Load Centered/X Load Position LADRC 2nd Order ==
  y : Inport
  r : Inport  Port=2
  Constant : Constant
  Demux : Demux  Outputs=3
  Divide : Product  Inputs=*/
  Gain1 : Gain  Gain=2
  Integrator : Integrator  InitialCondition=[0 0 0]'
  LESO : MATLAB Function  TreatAsAtomicUnit=on
  Product : Product
  Product1 : Product
  Saturation : Saturate  UpperLimit=10  LowerLimit=-10
  Square : Math  Operator=square
  Sum1 : Sum  Inputs=+-|
  Sum2 : Sum  Inputs=|+-
  Sum3 : Sum  Inputs=+-|
  b1 : Gain  Gain=b
  bw_c1 : Gain  Gain=bw_con
  bw_o1 : Gain  Gain=bw_eso
  u : Outport
  wires:
  LESO/1(z_dot) -> Integrator/1
  Integrator/1 -> LESO/1(z), Demux/1
  Demux/1 -> Sum3/2  "z1"
  Product/1 -> Sum1/1
  Sum1/1 -> Sum2/1  "u_0"
  Demux/3 -> Sum2/2  "z3"
  Sum2/1 -> Divide/1
  Square/1 -> Product/1
  Gain1/1 -> Product1/1
  Demux/2 -> Product1/2  "z2"
  Product1/1 -> Sum1/2
  r/1 -> Sum3/1
  Sum3/1 -> Product/2
  b1/1 -> Divide/2, LESO/3(b)
  bw_c1/1 -> Gain1/1, Square/1
  bw_o1/1 -> LESO/2(wo)
  y/1 -> LESO/4(y)
  Constant/1 -> bw_o1/1, bw_c1/1, b1/1
  Divide/1 -> Saturation/1  "u"
  Saturation/1 -> LESO/5(u), u/1

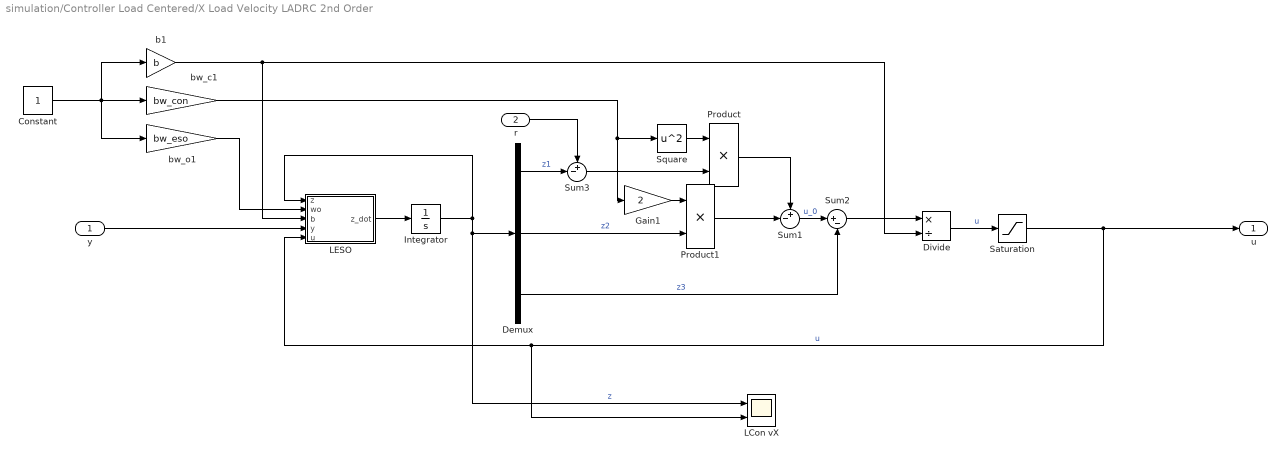
== system simulation/Controller Load Centered/X Load Velocity LADRC 2nd Order ==
  y : Inport
  r : Inport  Port=2
  Constant : Constant
  Demux : Demux  Outputs=3
  Divide : Product  Inputs=*/
  Gain1 : Gain  Gain=2
  Integrator : Integrator  InitialCondition=[0 0 0]'
  LCon vX : Scope  NumInputPorts=2
  LESO : MATLAB Function  TreatAsAtomicUnit=on
  Product : Product
  Product1 : Product
  Saturation : Saturate  UpperLimit=ldx_sat(2)  LowerLimit=ldx_sat(1)
  Square : Math  Operator=square
  Sum1 : Sum  Inputs=+-|
  Sum2 : Sum  Inputs=|+-
  Sum3 : Sum  Inputs=+-|
  b1 : Gain  Gain=b
  bw_c1 : Gain  Gain=bw_con
  bw_o1 : Gain  Gain=bw_eso
  u : Outport
  wires:
  LESO/1(z_dot) -> Integrator/1
  Integrator/1 -> LESO/1(z), LCon vX/1, Demux/1  "z"
  Demux/1 -> Sum3/2  "z1"
  Product/1 -> Sum1/1
  Sum1/1 -> Sum2/1  "u_0"
  Demux/3 -> Sum2/2  "z3"
  Sum2/1 -> Divide/1
  Square/1 -> Product/1
  Gain1/1 -> Product1/1
  Demux/2 -> Product1/2  "z2"
  Product1/1 -> Sum1/2
  r/1 -> Sum3/1
  Sum3/1 -> Product/2
  b1/1 -> Divide/2, LESO/3(b)
  bw_c1/1 -> Gain1/1, Square/1
  bw_o1/1 -> LESO/2(wo)
  y/1 -> LESO/4(y)
  Constant/1 -> bw_o1/1, bw_c1/1, b1/1
  Divide/1 -> Saturation/1  "u"
  Saturation/1 -> LCon vX/2, LESO/5(u), u/1  "u"

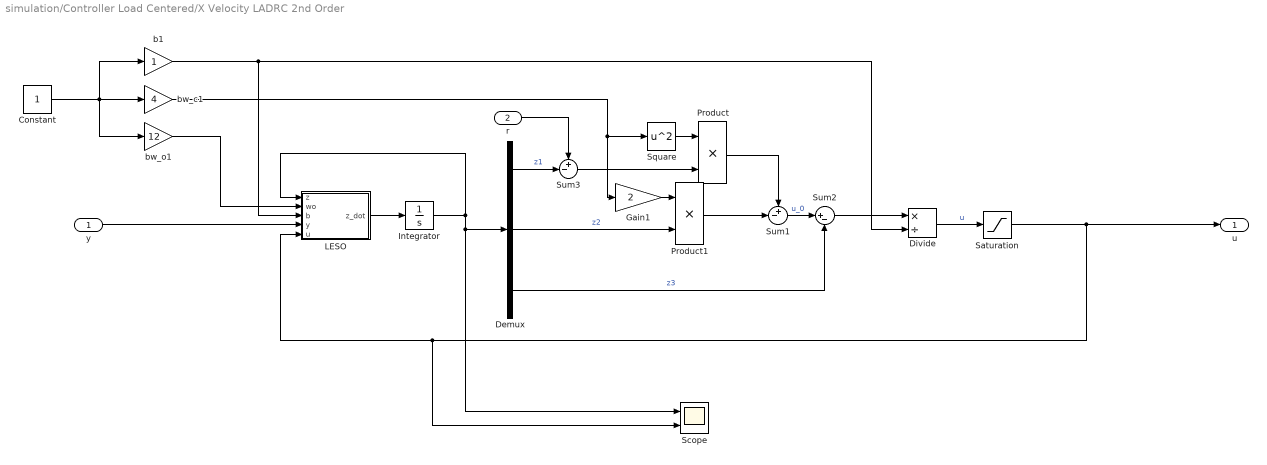
== system simulation/Controller Load Centered/X Velocity LADRC 2nd Order ==
  y : Inport
  r : Inport  Port=2
  Constant : Constant
  Demux : Demux  Outputs=3
  Divide : Product  Inputs=*/
  Gain1 : Gain  Gain=2
  Integrator : Integrator  InitialCondition=[0 0 0]'
  LESO : MATLAB Function  TreatAsAtomicUnit=on
  Product : Product
  Product1 : Product
  Saturation : Saturate  UpperLimit=xyforce(2)  LowerLimit=xyforce(1)
  Scope : Scope  NumInputPorts=2
  Square : Math  Operator=square
  Sum1 : Sum  Inputs=+-|
  Sum2 : Sum  Inputs=|+-
  Sum3 : Sum  Inputs=+-|
  b1 : Gain
  bw_c1 : Gain  Gain=4
  bw_o1 : Gain  Gain=12
  u : Outport
  wires:
  LESO/1(z_dot) -> Integrator/1
  Integrator/1 -> LESO/1(z), Scope/1, Demux/1
  Demux/1 -> Sum3/2  "z1"
  Product/1 -> Sum1/1
  Sum1/1 -> Sum2/1  "u_0"
  Demux/3 -> Sum2/2  "z3"
  Sum2/1 -> Divide/1
  Square/1 -> Product/1
  Gain1/1 -> Product1/1
  Demux/2 -> Product1/2  "z2"
  Product1/1 -> Sum1/2
  r/1 -> Sum3/1
  Sum3/1 -> Product/2
  b1/1 -> Divide/2, LESO/3(b)
  bw_c1/1 -> Gain1/1, Square/1
  bw_o1/1 -> LESO/2(wo)
  y/1 -> LESO/4(y)
  Constant/1 -> bw_o1/1, bw_c1/1, b1/1
  Divide/1 -> Saturation/1  "u"
  Saturation/1 -> Scope/2, LESO/5(u), u/1

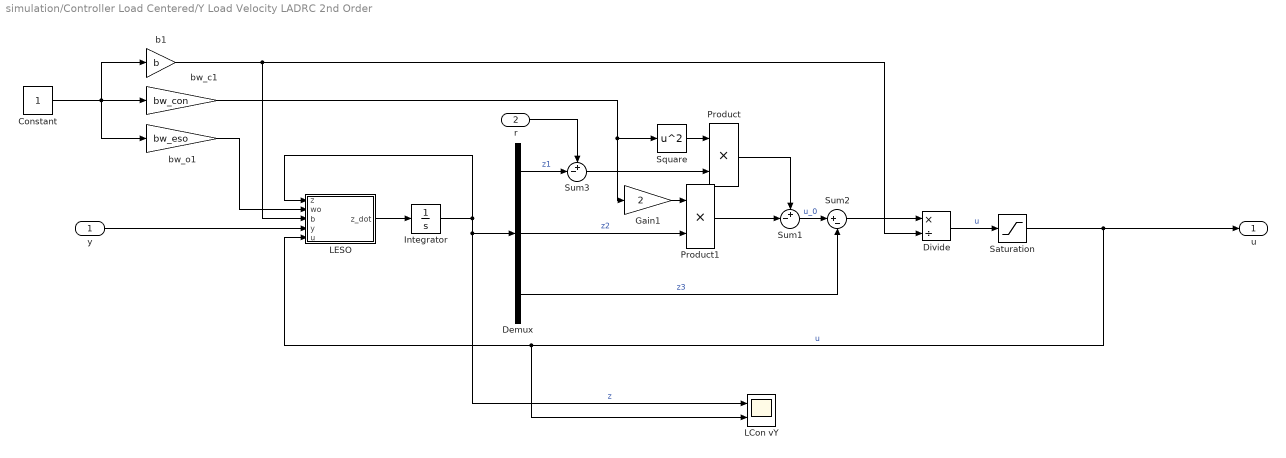
== system simulation/Controller Load Centered/Y Load Velocity LADRC 2nd Order ==
  y : Inport
  r : Inport  Port=2
  Constant : Constant
  Demux : Demux  Outputs=3
  Divide : Product  Inputs=*/
  Gain1 : Gain  Gain=2
  Integrator : Integrator  InitialCondition=[0 0 0]'
  LCon vY : Scope  NumInputPorts=2
  LESO : MATLAB Function  TreatAsAtomicUnit=on
  Product : Product
  Product1 : Product
  Saturation : Saturate  UpperLimit=ldy_sat(2)  LowerLimit=ldy_sat(1)
  Square : Math  Operator=square
  Sum1 : Sum  Inputs=+-|
  Sum2 : Sum  Inputs=|+-
  Sum3 : Sum  Inputs=+-|
  b1 : Gain  Gain=b
  bw_c1 : Gain  Gain=bw_con
  bw_o1 : Gain  Gain=bw_eso
  u : Outport
  wires:
  LESO/1(z_dot) -> Integrator/1
  Integrator/1 -> LESO/1(z), LCon vY/1, Demux/1  "z"
  Demux/1 -> Sum3/2  "z1"
  Product/1 -> Sum1/1
  Sum1/1 -> Sum2/1  "u_0"
  Demux/3 -> Sum2/2  "z3"
  Sum2/1 -> Divide/1
  Square/1 -> Product/1
  Gain1/1 -> Product1/1
  Demux/2 -> Product1/2  "z2"
  Product1/1 -> Sum1/2
  r/1 -> Sum3/1
  Sum3/1 -> Product/2
  b1/1 -> Divide/2, LESO/3(b)
  bw_c1/1 -> Gain1/1, Square/1
  bw_o1/1 -> LESO/2(wo)
  y/1 -> LESO/4(y)
  Constant/1 -> bw_o1/1, bw_c1/1, b1/1
  Divide/1 -> Saturation/1  "u"
  Saturation/1 -> LCon vY/2, LESO/5(u), u/1  "u"

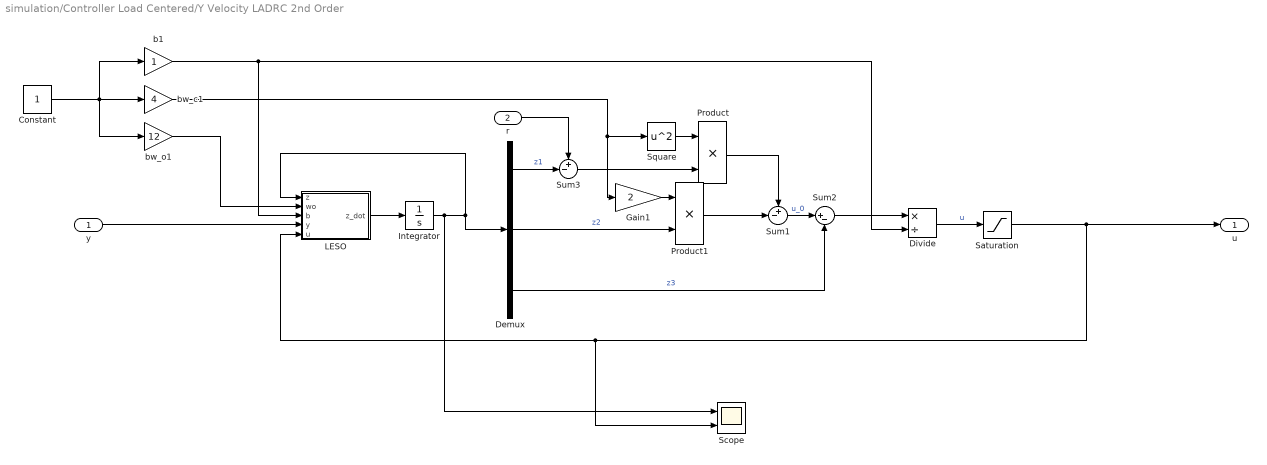
== system simulation/Controller Load Centered/Y Velocity LADRC 2nd Order ==
  y : Inport
  r : Inport  Port=2
  Constant : Constant
  Demux : Demux  Outputs=3
  Divide : Product  Inputs=*/
  Gain1 : Gain  Gain=2
  Integrator : Integrator  InitialCondition=[0 0 0]'
  LESO : MATLAB Function  TreatAsAtomicUnit=on
  Product : Product
  Product1 : Product
  Saturation : Saturate  UpperLimit=xyforce(2)  LowerLimit=xyforce(1)
  Scope : Scope  NumInputPorts=2
  Square : Math  Operator=square
  Sum1 : Sum  Inputs=+-|
  Sum2 : Sum  Inputs=|+-
  Sum3 : Sum  Inputs=+-|
  b1 : Gain
  bw_c1 : Gain  Gain=4
  bw_o1 : Gain  Gain=12
  u : Outport
  wires:
  LESO/1(z_dot) -> Integrator/1
  Integrator/1 -> Scope/1, LESO/1(z), Demux/1
  Demux/1 -> Sum3/2  "z1"
  Product/1 -> Sum1/1
  Sum1/1 -> Sum2/1  "u_0"
  Demux/3 -> Sum2/2  "z3"
  Sum2/1 -> Divide/1
  Square/1 -> Product/1
  Gain1/1 -> Product1/1
  Demux/2 -> Product1/2  "z2"
  Product1/1 -> Sum1/2
  r/1 -> Sum3/1
  Sum3/1 -> Product/2
  b1/1 -> Divide/2, LESO/3(b)
  bw_c1/1 -> Gain1/1, Square/1
  bw_o1/1 -> LESO/2(wo)
  y/1 -> LESO/4(y)
  Constant/1 -> bw_o1/1, bw_c1/1, b1/1
  Divide/1 -> Saturation/1  "u"
  Saturation/1 -> Scope/2, LESO/5(u), u/1

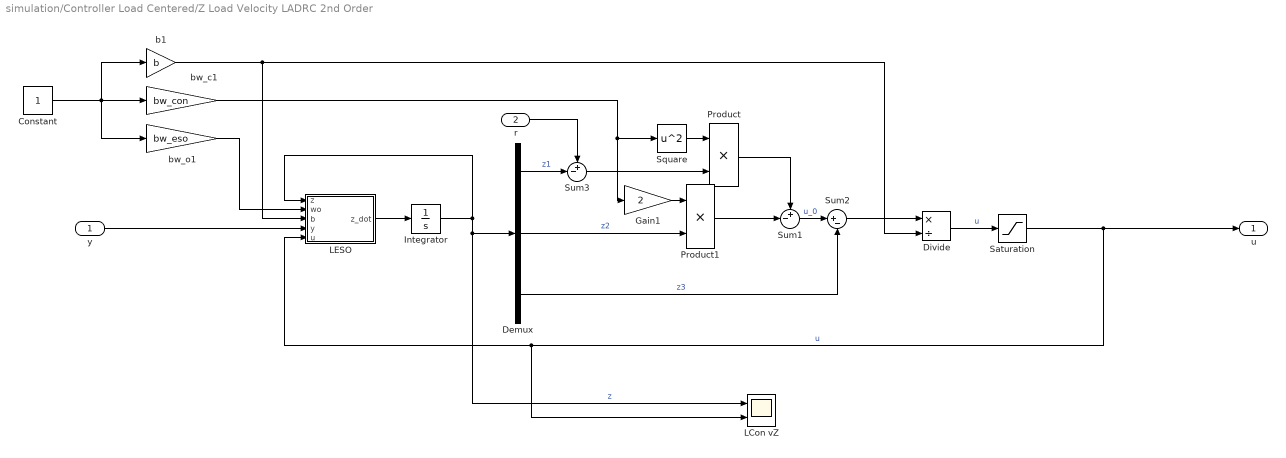
== system simulation/Controller Load Centered/Z Load Velocity LADRC 2nd Order ==
  y : Inport
  r : Inport  Port=2
  Constant : Constant
  Demux : Demux  Outputs=3
  Divide : Product  Inputs=*/
  Gain1 : Gain  Gain=2
  Integrator : Integrator  InitialCondition=[0 0 0]'
  LCon vZ : Scope  NumInputPorts=2
  LESO : MATLAB Function  TreatAsAtomicUnit=on
  Product : Product
  Product1 : Product
  Saturation : Saturate  UpperLimit=ldz_sat(2)  LowerLimit=ldz_sat(1)
  Square : Math  Operator=square
  Sum1 : Sum  Inputs=+-|
  Sum2 : Sum  Inputs=|+-
  Sum3 : Sum  Inputs=+-|
  b1 : Gain  Gain=b
  bw_c1 : Gain  Gain=bw_con
  bw_o1 : Gain  Gain=bw_eso
  u : Outport
  wires:
  LESO/1(z_dot) -> Integrator/1
  Integrator/1 -> LESO/1(z), LCon vZ/1, Demux/1  "z"
  Demux/1 -> Sum3/2  "z1"
  Product/1 -> Sum1/1
  Sum1/1 -> Sum2/1  "u_0"
  Demux/3 -> Sum2/2  "z3"
  Sum2/1 -> Divide/1
  Square/1 -> Product/1
  Gain1/1 -> Product1/1
  Demux/2 -> Product1/2  "z2"
  Product1/1 -> Sum1/2
  r/1 -> Sum3/1
  Sum3/1 -> Product/2
  b1/1 -> Divide/2, LESO/3(b)
  bw_c1/1 -> Gain1/1, Square/1
  bw_o1/1 -> LESO/2(wo)
  y/1 -> LESO/4(y)
  Constant/1 -> bw_o1/1, bw_c1/1, b1/1
  Divide/1 -> Saturation/1  "u"
  Saturation/1 -> LCon vZ/2, LESO/5(u), u/1  "u"

== system simulation/Controller Load Centered/Z Velocity LADRC 2nd Order ==
  y : Inport
  r : Inport  Port=2
  Constant : Constant
  Demux : Demux  Outputs=3
  Divide : Product  Inputs=*/
  Gain1 : Gain  Gain=2
  Integrator : Integrator  InitialCondition=[0 0 0]'
  LESO : MATLAB Function  TreatAsAtomicUnit=on
  Product : Product
  Product1 : Product
  Saturation : Saturate  UpperLimit=zforce(2)  LowerLimit=zforce(1)
  Square : Math  Operator=square
  Sum1 : Sum  Inputs=+-|
  Sum2 : Sum  Inputs=|+-
  Sum3 : Sum  Inputs=+-|
  b1 : Gain
  bw_c1 : Gain  Gain=4
  bw_o1 : Gain  Gain=12
  u : Outport
  wires:
  LESO/1(z_dot) -> Integrator/1
  Integrator/1 -> LESO/1(z), Demux/1
  Demux/1 -> Sum3/2  "z1"
  Product/1 -> Sum1/1
  Sum1/1 -> Sum2/1  "u_0"
  Demux/3 -> Sum2/2  "z3"
  Sum2/1 -> Divide/1
  Square/1 -> Product/1
  Gain1/1 -> Product1/1
  Demux/2 -> Product1/2  "z2"
  Product1/1 -> Sum1/2
  r/1 -> Sum3/1
  Sum3/1 -> Product/2
  b1/1 -> Divide/2, LESO/3(b)
  bw_c1/1 -> Gain1/1, Square/1
  bw_o1/1 -> LESO/2(wo)
  y/1 -> LESO/4(y)
  Constant/1 -> bw_o1/1, bw_c1/1, b1/1
  Divide/1 -> Saturation/1  "u"
  Saturation/1 -> LESO/5(u), u/1

== matlab function simulation/Controller Load Centered/X Load Velocity LADRC 2nd Order/LESO ==
  data: z input; wo input; b input; z_dot output; y input; u input
function z_dot = LESO(z, wo, b, y, u)
    A = [0 1 0; 0 0 1; 0 0 0];
    B = [0 b 0]';
    C = [1 0 0];
    L = [3*wo 3*wo^2 wo^3]';
        
    z_dot = (A*z + B*u + L*(y-C*z));

== matlab function simulation/Controller Load Centered/X Velocity LADRC 2nd Order/LESO ==
  data: z input; wo input; b input; z_dot output; y input; u input
function z_dot = LESO(z, wo, b, y, u)
    A = [0 1 0; 0 0 1; 0 0 0];
    B = [0 b 0]';
    C = [1 0 0];
    L = [3*wo 3*wo^2 wo^3]';
        
    z_dot = (A*z + B*u + L*(y-C*z));

== matlab function simulation/Controller Load Centered/Y Load Velocity LADRC 2nd Order/LESO ==
  data: z input; wo input; b input; z_dot output; y input; u input
function z_dot = LESO(z, wo, b, y, u)
    A = [0 1 0; 0 0 1; 0 0 0];
    B = [0 b 0]';
    C = [1 0 0];
    L = [3*wo 3*wo^2 wo^3]';
        
    z_dot = (A*z + B*u + L*(y-C*z));

== matlab function simulation/Controller Load Centered/Y Velocity LADRC 2nd Order/LESO ==
  data: z input; wo input; b input; z_dot output; y input; u input
function z_dot = LESO(z, wo, b, y, u)
    A = [0 1 0; 0 0 1; 0 0 0];
    B = [0 b 0]';
    C = [1 0 0];
    L = [3*wo 3*wo^2 wo^3]';
        
    z_dot = (A*z + B*u + L*(y-C*z));

== matlab function simulation/Plant/MATLAB Function ==
  data: nu input; eta input; u input; eta_d output; L parameter; m_l parameter; m_c parameter; g parameter; d parameter
function eta_d  = dynamics(nu, eta, u, L, m_l, m_c, g, d)

eta_d = zeros(5,1);

phi = nu(4);
theta = nu(5);

dphi = eta(4);
dtheta = eta(5);

M = [m_l+m_c,           0,                              0,                              0,                          L*m_l*cos(theta);
    0,                  m_l+m_c,                        0,                             -L*m_l*cos(phi)*cos(theta),  L*m_l*sin(phi)*sin(theta);
    0,                  0,                              m_l+m_c,                       -L*m_l*cos(theta)*sin(phi), -L*m_l*cos(phi)*sin(theta);
    0,                 -L*m_l*cos(phi)*cos(theta),     -L*m_l*cos(theta)*sin(phi),      L^2*m_l*cos(theta)^2,       0;
    L*m_l*cos(theta),   L*m_l*sin(phi)*sin(theta),     -L*m_l*cos(phi)*sin(theta),      0,                          L^2*m_l];
% M_i = inv(M);

C = [0, 0, 0,  0,                                                                           -L*dtheta*m_l*sin(theta);
     0, 0, 0,  L*m_l*(dphi*cos(theta)*sin(phi)+dtheta*cos(phi)*sin(theta)),      L*m_l*(dphi*cos(phi)*sin(theta)+dtheta*cos(theta)*sin(phi));
     0, 0, 0, -L*m_l*(dphi*cos(phi)*cos(theta)-dtheta*sin(phi)*sin(theta)),     -L*m_l*(dtheta*cos(phi)*cos(theta)-dphi*sin(phi)*sin(theta));
     0, 0, 0, -0.5*L^2*dtheta*m_l*sin(2*theta),                                        -0.5*L^2*dphi*m_l*sin(2*theta);
     0, 0, 0,  0.5*L^2*dphi*m_l*sin(2*theta), 0];

G = [0;
     0;
     -g*(m_l + m_c);
      L*g*m_l*cos(theta)*sin(phi);
      L*g*m_l*cos(phi)*sin(theta)];
D = diag([0, 0, 0, d, d]);

% To protect against singularities
epsilon = 0.0001;
M(4,4) = L^2*m_l*cos(theta)^2 + epsilon*sin(theta)^2;
C(4,4) = -0.5*L^2*m_l*dtheta*sin(2*theta)+0.5*epsilon*dtheta*sin(2*theta);

eta_d = M\([u; 0; 0;] - C*eta - G - D*eta);

== matlab function simulation/Controller Load Centered/Z Load Velocity LADRC 2nd Order/LESO ==
  data: z input; wo input; b input; z_dot output; y input; u input
function z_dot = LESO(z, wo, b, y, u)
    A = [0 1 0; 0 0 1; 0 0 0];
    B = [0 b 0]';
    C = [1 0 0];
    L = [3*wo 3*wo^2 wo^3]';
        
    z_dot = (A*z + B*u + L*(y-C*z));

== matlab function simulation/Controller Load Centered/Z Velocity LADRC 2nd Order/LESO ==
  data: z input; wo input; b input; z_dot output; y input; u input
function z_dot = LESO(z, wo, b, y, u)
    A = [0 1 0; 0 0 1; 0 0 0];
    B = [0 b 0]';
    C = [1 0 0];
    L = [3*wo 3*wo^2 wo^3]';
        
    z_dot = (A*z + B*u + L*(y-C*z));

== matlab function simulation/Controller Drone Centered/Y Velocity LADRC 2nd Order/LESO ==
  data: z input; wo input; b input; z_dot output; y input; u input
function z_dot = LESO(z, wo, b, y, u)
    A = [0 1 0; 0 0 1; 0 0 0];
    B = [0 b 0]';
    C = [1 0 0];
    L = [3*wo 3*wo^2 wo^3]';
        
    z_dot = (A*z + B*u + L*(y-C*z));

== matlab function simulation/Controller Drone Centered/X Velocity LADRC 2nd Order/LESO ==
  data: z input; wo input; b input; z_dot output; y input; u input
function z_dot = LESO(z, wo, b, y, u)
    A = [0 1 0; 0 0 1; 0 0 0];
    B = [0 b 0]';
    C = [1 0 0];
    L = [3*wo 3*wo^2 wo^3]';
        
    z_dot = (A*z + B*u + L*(y-C*z));

== matlab function simulation/Controller Drone Centered/Z Velocity LADRC 2nd Order/LESO ==
  data: z input; wo input; b input; z_dot output; y input; u input
function z_dot = LESO(z, wo, b, y, u)
    A = [0 1 0; 0 0 1; 0 0 0];
    B = [0 b 0]';
    C = [1 0 0];
    L = [3*wo 3*wo^2 wo^3]';
        
    z_dot = (A*z + B*u + L*(y-C*z));

== matlab function simulation/Navigation/MATLAB Function ==
  data: pos output; vect output; x input; y input; z input; phi input; theta input; L parameter
function [pos,vect]  = fcn(x, y, z, phi, theta, L)
    R_x = [1 0        0;
           0 cos(phi) -sin(phi);
           0 sin(phi) cos(phi)];
%     R_y = [cos(theta)  0 sin(theta);
%            0           1 0;
%            -sin(theta) 0 cos(theta)];
    R_y = [cos(-theta)  0 sin(-theta);
           0           1 0;
           -sin(-theta) 0 cos(-theta)];
    R = R_x * R_y;

vect = [0 0 1]';

vect = R*vect;
pos = [x y z]'+L*vect;

== matlab function simulation/Navigation/MATLAB Function1 ==
  data: x input; y input; norm output; z input
function norm= fcn(x, y, z)

norm = sqrt(x*x + y*y + z*z);

== matlab function simulation/Plant/Load Polar to Cartesian ==
  data: q input; pos output; qd input; qdd input; vel output; acc output; L parameter
function [pos, vel, acc] = fcn(q, qd, qdd, L)

x = q(1);
y = q(2);
z = q(3);
phi = q(4);
theta = q(5);

dx = qd(1);
dy = qd(2);
dz = qd(3);
dphi = qd(4);
dtheta = qd(5);

ddx = qdd(1);
ddy = qdd(2);
ddz = qdd(3);
ddphi = qdd(4);
ddtheta = qdd(5);


pos = [x + L*sin(theta) ;
        y - L*cos(theta)*sin(phi);
        z + L*cos(theta)*cos(phi);
        phi;
        theta]';

vel = [dx + L*dtheta*cos(theta);
        dy + L*(dtheta*sin(theta)*sin(phi) - dphi*cos(theta)*cos(phi));
        dz - L*(dtheta*sin(theta)*cos(phi) + dphi*cos(theta)*sin(phi));
        dphi;
        dtheta]';

% WRONG
% pos = [x - L*sin(theta) ;
%         y - L*cos(theta)*sin(phi);
%         z + L*cos(theta)*cos(phi);
%         phi;
%         theta]';


% WRONG
% vel = [dx - L*dtheta*cos(theta);
%         dy + L*(dtheta*sin(theta)*sin(phi) - dphi*cos(theta)*cos(phi));
%         dz - L*(dtheta*cos(theta)*sin(phi) - dphi*sin(theta)*cos(phi));
%         dphi;
%         dtheta]';

acc = [ddx - L*(ddtheta*cos(theta) - dtheta^2*sin(theta));
        ddy + L*(ddtheta*sin(theta)*sin(phi) - ddphi*cos(theta)*cos(phi) + (dtheta^2 + dphi^2)*cos(theta)*sin(phi) + 2*dtheta*dphi*sin(theta)*cos(phi));
        ddz - L*(ddtheta*sin(theta)*cos(phi) + ddphi*cos(theta)*sin(phi) + (dtheta^2 + dphi^2)*cos(theta)*cos(phi) - 2*dtheta*dphi*sin(theta)*sin(phi));
        ddphi;
        ddtheta]';

== matlab function simulation/Controller Load Centered/X Load Position LADRC 2nd Order/LESO ==
  data: z input; wo input; b input; z_dot output; y input; u input
function z_dot = LESO(z, wo, b, y, u)
    A = [0 1 0; 0 0 1; 0 0 0];
    B = [0 b 0]';
    C = [1 0 0];
    L = [3*wo 3*wo^2 wo^3]';
        
    z_dot = (A*z + B*u + L*(y-C*z));
